simulink model "TestBateria"  (R2023b)
settings: Solver=VariableStepAuto  StartTime=0.0  StopTime=inf  RelTol=1e-3
libraries: arduinolib x1
settings Model: Creator=Usuario_UMA  LastModifiedBy=Diego

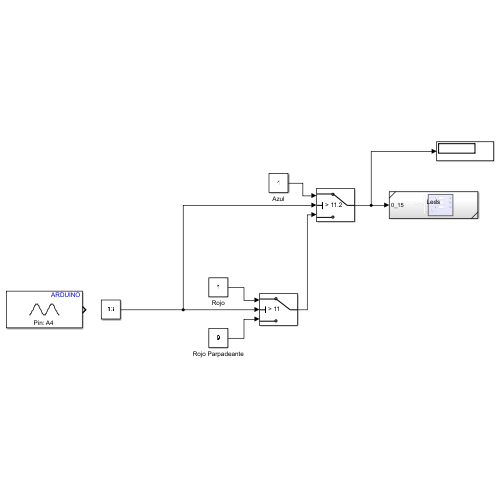
[thumbnail: Simulink's stored preview of the top-level diagram]
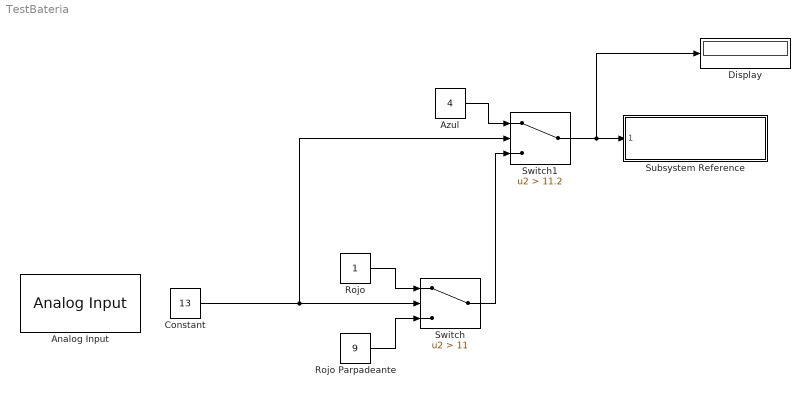
== system TestBateria ==
  Analog Input : arduinolib/Analog Input  pinNumber=4  ReadResultsOnly=off  ConversionTriggerSource=Software  ExternalTriggerType=uint32( 0 )  OutputDataType=uint16  EnableConversionCompleteNotify=off  EnableOuputStatus=off  SampleTime=-1  blockPlatform=arduino
  Azul : Constant  Value=4
  Constant : Constant  Value=13
  Display : Display
  Rojo : Constant
  Rojo Parpadeante : Constant  Value=9
  Subsystem Reference : Subsystem  ReferencedSubsystem=Leds
  Switch : Switch  Criteria=u2 > Threshold  Threshold=11  SaturateOnIntegerOverflow=off  InputSameDT=off
  Switch1 : Switch  Criteria=u2 > Threshold  Threshold=11.2  SaturateOnIntegerOverflow=off  InputSameDT=off
  wires:
  Switch1/1 -> Display/1, Subsystem Reference/1
  Constant/1 -> Switch1/2, Switch/2
  Azul/1 -> Switch1/1
  Rojo Parpadeante/1 -> Switch/3
  Rojo/1 -> Switch/1
  Switch/1 -> Switch1/3
